simulink model "mcb_pmsm_foc_sensorless_f28379d"  (R2024b)
settings: Solver=FixedStepDiscrete  StartTime=0.0  StopTime=8  RelTol=1e-3  EnableMultiTasking=on
InitFcn:
  | mcb_pmsm_foc_sensorless_f28379d_datascript;
model workspace (MAT data in the model file):
  encoderResolution = 2000
  hallOffset = '0.5'
  indexOffset = 850
  polePairs = '4'
values from neighbouring files (symbols this model uses):
  acceleration = 10000/PU_System.N_base    [mcb_pmsm_foc_sensorless_f28069MLaunchPad_edit_datascript.m]    (also in mcb_pmsm_foc_sensorless_f28379d_datascript.m)
  dataType = 'single'    [mcb_pmsm_foc_sensorless_f28069MLaunchPad_edit_datascript.m]    (also in mcb_pmsm_foc_sensorless_f28379d_datascript.m)
  inverter = mcb_SetInverterParameters('BoostXL-DRV8305')    [mcb_pmsm_foc_sensorless_f28069MLaunchPad_edit_datascript.m]    (also in mcb_pmsm_foc_sensorless_f28379d_datascript.m = mcb_updateInverterParameters(pmsm,inverter,target))
  MAX_OL_NEG_SPD = -0.2    [mcb_pmsm_foc_sensorless_f28069MLaunchPad_edit_datascript.m]    (also in mcb_pmsm_foc_sensorless_f28379d_datascript.m)
  MAX_OL_POS_SPD = 0.2    [mcb_pmsm_foc_sensorless_f28069MLaunchPad_edit_datascript.m]    (also in mcb_pmsm_foc_sensorless_f28379d_datascript.m)
  MAX_OL_VD_LIMIT = 0.6    [mcb_pmsm_foc_sensorless_f28069MLaunchPad_edit_datascript.m]    (also in mcb_pmsm_foc_sensorless_f28379d_datascript.m)
  MIN_CL_NEG_SPD = -0.15    [mcb_pmsm_foc_sensorless_f28069MLaunchPad_edit_datascript.m]    (also in mcb_pmsm_foc_sensorless_f28379d_datascript.m)
  MIN_CL_POS_SPD = 0.15    [mcb_pmsm_foc_sensorless_f28069MLaunchPad_edit_datascript.m]    (also in mcb_pmsm_foc_sensorless_f28379d_datascript.m)
  MIN_OL_VD_LIMIT = 0.15    [mcb_pmsm_foc_sensorless_f28069MLaunchPad_edit_datascript.m]    (also in mcb_pmsm_foc_sensorless_f28379d_datascript.m)
  one_sec_tick = uint16(1/Ts_speed)    [mcb_pmsm_foc_sensorless_f28069MLaunchPad_edit_datascript.m]    (also in mcb_pmsm_foc_sensorless_f28379d_datascript.m)
  PI_params = mcb_SetControllerParameters(pmsm,inverter,PU_System,T_pwm,2*Ts,2*Ts_speed)    [mcb_pmsm_foc_sensorless_f28069MLaunchPad_edit_datascript.m]    (also in mcb_pmsm_foc_sensorless_f28379d_datascript.m)
  pmsm = mcb_SetPMSMMotorParameters('BLY172S')    [mcb_pmsm_foc_sensorless_f28069MLaunchPad_edit_datascript.m]    (also in mcb_pmsm_foc_sensorless_f28379d_datascript.m)
  PU_System = mcb_SetPUSystem(pmsm,inverter)    [mcb_pmsm_foc_sensorless_f28069MLaunchPad_edit_datascript.m]    (also in mcb_pmsm_foc_sensorless_f28379d_datascript.m)
  RAMP_STEP_SIZE = 0.001    [mcb_pmsm_foc_sensorless_f28069MLaunchPad_edit_datascript.m]    (also in mcb_pmsm_foc_sensorless_f28379d_datascript.m)
  Speed_openLoop_PU = 0.1    [mcb_pmsm_foc_sensorless_f28069MLaunchPad_edit_datascript.m]    (also in mcb_pmsm_foc_sensorless_f28379d_datascript.m)
  target = mcb_SetProcessorDetails('F28069M',PWM_frequency)    [mcb_pmsm_foc_sensorless_f28069MLaunchPad_edit_datascript.m]    (also in mcb_pmsm_foc_sensorless_f28379d_datascript.m = mcb_SetProcessorDetails('F28379D',PWM_frequency))
  Ts = T_pwm    (= 5e-05)    [mcb_pmsm_foc_sensorless_f28069MLaunchPad_edit_datascript.m]    (also in mcb_pmsm_foc_sensorless_f28379d_datascript.m)
  Ts_motor = T_pwm/2    (= 2.5e-05)    [mcb_pmsm_foc_sensorless_f28069MLaunchPad_edit_datascript.m]    (also in mcb_pmsm_foc_sensorless_f28379d_datascript.m)
  Ts_simulink = T_pwm/2    (= 2.5e-05)    [mcb_pmsm_foc_sensorless_f28069MLaunchPad_edit_datascript.m]    (also in mcb_pmsm_foc_sensorless_f28379d_datascript.m)
  Ts_speed = 10*Ts    (= 0.0005)    [mcb_pmsm_foc_sensorless_f28069MLaunchPad_edit_datascript.m]    (also in mcb_pmsm_foc_sensorless_f28379d_datascript.m)
  two_sec_tick = uint16(2/Ts_speed)    [mcb_pmsm_foc_sensorless_f28069MLaunchPad_edit_datascript.m]    (also in mcb_pmsm_foc_sensorless_f28379d_datascript.m)
undefined symbols (not defined in the file or in its folder): Down, GPTRIP1SEL, GPTRIP2SEL, TZ1, TZ2, Up
libraries: mcbcontrolslib x17, simulink x8, c2802xlib x7, c280xlib x5, c2837xDlib x4, slpidlib x3, mcbpositiondecoderlib x3, mcbsensorlessestimatorlib x2, svdschedulerlib x2, svdutilitieslib x1, mcbplantlib x1, autolibpmsmexterior x1
(part 3 of 3)

== system mcb_pmsm_foc_sensorless_f28379d/Hardware Init/Variant Subsystem/Code Generation/Calculate ADC Offset  ==
  Enable : EnablePort
  Constant : Constant  Value=8
  Constant1 : Constant  Value=inverter.CtSensOffsetMax  OutDataTypeStr=Inherit: Inherit via back propagation
  Constant2 : Constant  Value=inverter.CtSensOffsetMin  OutDataTypeStr=Inherit: Inherit via back propagation
  Divide : Product  Inputs=*/  OutDataTypeStr=uint16
  Divide1 : Product  Inputs=*/  OutDataTypeStr=uint16
  For Iterator Subsystem : Subsystem  TreatAsAtomicUnit=on
  If : If  NumInputs=3  IfExpression=u1 > u3 & u1 < u2
  If Action Subsystem : Subsystem  TreatAsAtomicUnit=on
  If Action Subsystem1 : Subsystem  TreatAsAtomicUnit=on
  If Action Subsystem2 : Subsystem  TreatAsAtomicUnit=on
  If Action Subsystem3 : Subsystem  TreatAsAtomicUnit=on
  If1 : If  NumInputs=3  IfExpression=u1 > u3 & u1 < u2
  wires:
  For Iterator Subsystem/2(Out2) -> Divide1/1
  Divide/1 -> If Action Subsystem/1(In1), If/1
  For Iterator Subsystem/1(Out1) -> Divide/1
  Constant/1 -> Divide1/2, Divide/2
  Divide1/1 -> If Action Subsystem2/1(In1), If1/1
  If/1 -> If Action Subsystem/Action
  If/2 -> If Action Subsystem1/Action
  If1/1 -> If Action Subsystem2/Action
  If1/2 -> If Action Subsystem3/Action
  Constant1/1 -> If1/2, If/2
  Constant2/1 -> If/3, If1/3

== system mcb_pmsm_foc_sensorless_f28379d/Hardware Init/Variant Subsystem/Code Generation/DRV Enable ==
  note: Enable inverter in CPU1
  In : Inport
  ADC Gain Setting : Subsystem
  Constant : Constant  Value=inverter.EnableLogic
  Digital Output : c2837xDlib/Digital Output  Priority=10  GPIO_Number=GPIO120~GPIO127  GPIO_Bit0=off  GPIO_BIT0_Toggle=off  GPIO_Bit1=off  GPIO_BIT1_Toggle=off  GPIO_Bit2=off  GPIO_BIT2_Toggle=off  GPIO_Bit3=off  GPIO_BIT3_Toggle=off  GPIO_Bit4=on  GPIO_BIT4_Toggle=off  GPIO_Bit5=off  GPIO_BIT5_Toggle=off  GPIO_Bit6=off  GPIO_BIT6_Toggle=off  GPIO_Bit7=off  GPIO_BIT7_Toggle=off
  Digital Output1 : c2837xDlib/Digital Output  Priority=10  GPIO_Number=GPIO16~GPIO23  GPIO_Bit0=off  GPIO_BIT0_Toggle=off  GPIO_Bit1=off  GPIO_BIT1_Toggle=off  GPIO_Bit2=off  GPIO_BIT2_Toggle=off  GPIO_Bit3=off  GPIO_BIT3_Toggle=off  GPIO_Bit4=off  GPIO_BIT4_Toggle=off  GPIO_Bit5=off  GPIO_BIT5_Toggle=off  GPIO_Bit6=on  GPIO_BIT6_Toggle=off  GPIO_Bit7=off  GPIO_BIT7_Toggle=off
  Inverter Enable : Constant  OutDataTypeStr=uint16  SampleTime=-1
  NOT : Logic  Operator=NOT  IconShape=distinctive  AllPortsSameDT=off  OutDataTypeStr=boolean
  RunTimeMeasurement : Constant  OutDataTypeStr=uint16  SampleTime=-1
  Switch : Switch  Criteria=u2 > Threshold  SaturateOnIntegerOverflow=off  InputSameDT=off
  wires:
  RunTimeMeasurement/1 -> Digital Output1/1
  NOT/1 -> Switch/3  "Active low logic for inverter enable"
  Inverter Enable/1 -> Switch/1, NOT/1  "Active high logic for inverter enable"
  Constant/1 -> ADC Gain Setting/Enable, Switch/2
  Switch/1 -> Digital Output/1
  In/1 -> ADC Gain Setting/1(In1)

== system mcb_pmsm_foc_sensorless_f28379d/Hardware Init/Variant Subsystem/Code Generation/Default ADC Offset ==
  Enable : EnablePort
  Constant : Constant  Value=inverter.CtSensAOffset  OutDataTypeStr=Inherit: Inherit via back propagation
  Constant1 : Constant  Value=inverter.CtSensBOffset  OutDataTypeStr=Inherit: Inherit via back propagation
  Data Store Write1 : DataStoreWrite  DataStoreName=IaOffset  IndexOptions=Index vector (dialog)  Indices=1  OutputSizes=1
  Data Store Write2 : DataStoreWrite  DataStoreName=IbOffset  IndexOptions=Index vector (dialog)  Indices=1  OutputSizes=1
  wires:
  Constant/1 -> Data Store Write1/1
  Constant1/1 -> Data Store Write2/1

== system mcb_pmsm_foc_sensorless_f28379d/Serial Receive/SCI_Rx/Code Generation/Data_Type_Fixed_Point ==
  SCI Receive : c280xlib/SCI Receive  sciModule=A  dataHead=''  headerCheckMaxCount=16  dataTail=''  dataType=uint32  dataLenOptions=Length via dialog  dataDim=2  maxDataLength=1  initValue=0  errOption=Output the last received value  errValue=0  sampleTime=-1  blockingMode=on  timeOut=0.00875  outputStatus=off
  Data : Outport
  wires:
  SCI Receive/1 -> Data/1

== system mcb_pmsm_foc_sensorless_f28379d/Serial Receive/SCI_Rx/Code Generation/Data_Type_Float ==
  SCI Receive : c280xlib/SCI Receive  sciModule=A  dataHead=''  headerCheckMaxCount=16  dataTail=''  dataType=single  dataLenOptions=Length via dialog  dataDim=2  maxDataLength=1  initValue=0  errOption=Output the last received value  errValue=0  sampleTime=-1  blockingMode=on  timeOut=0.00875  outputStatus=off
  Data : Outport
  wires:
  SCI Receive/1 -> Data/1

== system mcb_pmsm_foc_sensorless_f28379d/Serial Receive/SCI_Rx/Simulation/Data_Conditioning_Tx ==
  In1 : Inport
  In2 : Inport  Port=2
  Data_Type_Fixed_Point : Subsystem  VariantControl=~isequal(dataType, 'single')
  Data_Type_Float : Subsystem  VariantControl=isequal(dataType, 'single')
  Data : Outport

== system mcb_pmsm_foc_sensorless_f28379d/Serial Receive/SCI_Rx/Simulation/Parse ==
  Enable_PWM : Inport
  Debug_signals : Inport  Port=2
  Bitwise Operator : simulink/Logic and Bit Operations/Bitwise Operator  logicop=AND  UseBitMask=on  BitMask=hex2dec('0001')  BitMaskRealWorld=Stored Integer
  Bitwise Operator1 : simulink/Logic and Bit Operations/Bitwise Operator  logicop=AND  UseBitMask=on  BitMask=hex2dec('00F0')  BitMaskRealWorld=Stored Integer
  Shift Arithmetic1 : ArithShift  BitShiftNumber=-4
  Sum : Sum
  Data : Outport
  wires:
  Bitwise Operator/1 -> Sum/1
  Debug_signals/1 -> Shift Arithmetic1/1
  Sum/1 -> Data/1
  Shift Arithmetic1/1 -> Bitwise Operator1/1
  Enable_PWM/1 -> Bitwise Operator/1
  Bitwise Operator1/1 -> Sum/2

== system mcb_pmsm_foc_sensorless_f28379d/Current Control/Closed Loop/Open_Loop_Control/Accumulate1/Subsystem ==
  Input : Inport
  Enable : EnablePort
  Out1 : Outport  InitialOutput=0
  wires:
  Input/1 -> Out1/1

== system mcb_pmsm_foc_sensorless_f28379d/Current Control/Input Scaling/Calculate Phase Currents/Data_Type/Data_Type_Fixed_Point ==
  In1 : Inport
  Data Type Conversion : DataTypeConversion  OutDataTypeStr=fixdt(1,32,17)  ConvertRealWorld=Stored Integer (SI)  RndMeth=Simplest  SaturateOnIntegerOverflow=off
  Data Type Conversion1 : DataTypeConversion  OutDataTypeStr=dataType  RndMeth=Simplest  SaturateOnIntegerOverflow=off
  Q17 per unit conversion : ArithShift  BitShiftNumber=-6
  Iab_meas_PU : Outport
  wires:
  In1/1 -> Q17 per unit conversion/1
  Data Type Conversion1/1 -> Iab_meas_PU/1
  Data Type Conversion/1 -> Data Type Conversion1/1
  Q17 per unit conversion/1 -> Data Type Conversion/1

== system mcb_pmsm_foc_sensorless_f28379d/Current Control/Input Scaling/Calculate Phase Currents/Data_Type/Data_Type_Float ==
  In1 : Inport
  Get ADC Voltage : Gain  Gain=target.ADC_Vref /target.ADC_MaxCount  OutDataTypeStr=dataType  RndMeth=Simplest
  Get Currents : Gain  Gain=1/inverter.ISenseVoltPerAmp  RndMeth=Simplest  OutDataTypeStr=Inherit: Same as input
  PU_Conversion : Gain  Gain=1/PU_System.I_base  RndMeth=Simplest  OutDataTypeStr=Inherit: Same as input
  Iab_meas_PU : Outport
  wires:
  Get ADC Voltage/1 -> Get Currents/1
  Get Currents/1 -> PU_Conversion/1
  PU_Conversion/1 -> Iab_meas_PU/1
  In1/1 -> Get ADC Voltage/1

== system mcb_pmsm_foc_sensorless_f28379d/Current Control/Input Scaling/Calculate position and speed/Flux Observer/DC component removal ==
  SigIN : Inport
  IIR Filter : mcbcontrolslib/IIR Filter  VariantControl=Low Pass Filter  VariantSelect=High-pass  FilterConstantInputType=Specify via dialog  Filter_constant=0.0005*(Ts/50e-6)  advancedSettings=on  Ts=50e-6  cutOff_freq=1
  SigOUT : Outport
  wires:
  SigIN/1 -> IIR Filter/1
  IIR Filter/1 -> SigOUT/1

== system mcb_pmsm_foc_sensorless_f28379d/Current Control/Input Scaling/Calculate position and speed/Flux Observer/DC component removal1 ==
  SigIN : Inport
  IIR Filter : mcbcontrolslib/IIR Filter  VariantControl=Low Pass Filter  VariantSelect=Low-pass  FilterConstantInputType=Specify via dialog  Filter_constant=0.005*(Ts/50e-6)  advancedSettings=on  Ts=50e-6  cutOff_freq=1
  Sum6 : Sum  Inputs=|+-  RndMeth=Simplest  OutDataTypeStr=Inherit: Same as first input
  SigOUT : Outport
  wires:
  Sum6/1 -> SigOUT/1
  SigIN/1 -> Sum6/1, IIR Filter/1
  IIR Filter/1 -> Sum6/2

== system mcb_pmsm_foc_sensorless_f28379d/Current Control/SCI_Tx/Code Generation/Data_Conditioning_Tx/Data_Type_Fixed_Point ==
  In1 : Inport
  Data Type Conversion : DataTypeConversion  OutDataTypeStr=fixdt(1,32,28)  RndMeth=Simplest  SaturateOnIntegerOverflow=off
  Data Type Conversion3 : DataTypeConversion  OutDataTypeStr=uint32  ConvertRealWorld=Stored Integer (SI)  RndMeth=Simplest  SaturateOnIntegerOverflow=off
  Data_Log : Outport
  wires:
  In1/1 -> Data Type Conversion/1
  Data Type Conversion3/1 -> Data_Log/1
  Data Type Conversion/1 -> Data Type Conversion3/1

== system mcb_pmsm_foc_sensorless_f28379d/Current Control/SCI_Tx/Code Generation/Data_Conditioning_Tx/Data_Type_Float ==
  In1 : Inport
  Byte Pack : svdutilitieslib/Byte Pack  maskPackedDataType=uint32  datatypes={'single'}  byteAlign=4  blockPlatform=tic2000
  Data_Log : Outport
  wires:
  Byte Pack/1 -> Data_Log/1
  In1/1 -> Byte Pack/1

== system mcb_pmsm_foc_sensorless_f28379d/Current Control/SCI_Tx/Code Generation/Data_Logging/Data ==
  Data : Inport
  Data_width : Inport  Port=2
  Action Port : ActionPort  ActionPortLabel=else
  Dummy : Constant  Value=hex2dec('0000')  OutDataTypeStr=uint32
  Mux : Mux  Inputs=2
  Data_out : Outport  VectorParamsAs1DForOutWhenUnconnected=off
  Iteration : Outport  Port=2  VectorParamsAs1DForOutWhenUnconnected=off
  wires:
  Data_width/1 -> Iteration/1
  Data/1 -> Mux/1
  Dummy/1 -> Mux/2
  Mux/1 -> Data_out/1

== system mcb_pmsm_foc_sensorless_f28379d/Current Control/SCI_Tx/Code Generation/Data_Logging/End ==
  Data : Inport
  Data_width : Inport  Port=2
  Action Port : ActionPort  ActionPortLabel=elseif(u1 == 599)
  Bias : Bias  Bias=1  SaturateOnIntegerOverflow=off
  End : Constant  Value=hex2dec('45454545')  OutDataTypeStr=uint32
  Mux : Mux  Inputs=2
  Data_out : Outport  VectorParamsAs1DForOutWhenUnconnected=off
  Iteration : Outport  Port=2  VectorParamsAs1DForOutWhenUnconnected=off
  wires:
  Data/1 -> Mux/1
  Data_width/1 -> Bias/1
  Bias/1 -> Iteration/1
  End/1 -> Mux/2
  Mux/1 -> Data_out/1

== system mcb_pmsm_foc_sensorless_f28379d/Current Control/SCI_Tx/Code Generation/Data_Logging/Start ==
  Data : Inport
  Data_width : Inport  Port=2
  Action Port : ActionPort  ActionPortLabel=if(u1 == 0)
  Bias : Bias  Bias=1  SaturateOnIntegerOverflow=off
  Mux : Mux  Inputs=2
  Start : Constant  Value=hex2dec('53535353')  OutDataTypeStr=uint32
  Data_out : Outport  VectorParamsAs1DForOutWhenUnconnected=off
  Iteration : Outport  Port=2  VectorParamsAs1DForOutWhenUnconnected=off
  wires:
  Data/1 -> Mux/2
  Data_width/1 -> Bias/1
  Bias/1 -> Iteration/1
  Start/1 -> Mux/1
  Mux/1 -> Data_out/1

== system mcb_pmsm_foc_sensorless_f28379d/Hardware Init/Variant Subsystem/Code Generation/Calculate ADC Offset /For Iterator Subsystem ==
  ADC_B2 : c2802xlib/ADC  Priority=20  blkParamProc=C2000_Type4  ADCModule=B  samplingMode=Single sample mode  ADCResolution=12-bit (Single-ended input)  useSOC1=SOC2  useSOC2=SOC0_SOC1  SOCAcquisitionWindow=15  SOCTriggerSource=Software  SOCInterruptTrigger=No ADCINT  Ts=-1  dType=uint16  postInterrupt=off  interruptSel=ADCINT1  ADCINTContinuous=on  endma=off  chdma=1  conv1=ADCINA0  conv2=ADCINA0 and ADCINB0  conv1_Type4=ADCIN2  conv2_Type4=ADCIN0 and ADCIN1
  ADC_C2 : c2802xlib/ADC  Priority=20  blkParamProc=C2000_Type4  ADCModule=C  samplingMode=Single sample mode  ADCResolution=12-bit (Single-ended input)  useSOC1=SOC2  useSOC2=SOC0_SOC1  SOCAcquisitionWindow=15  SOCTriggerSource=Software  SOCInterruptTrigger=No ADCINT  Ts=-1  dType=uint16  postInterrupt=off  interruptSel=ADCINT1  ADCINTContinuous=on  endma=off  chdma=1  conv1=ADCINA0  conv2=ADCINA0 and ADCINB0  conv1_Type4=ADCIN2  conv2_Type4=ADCIN0 and ADCIN1
  For Iterator : ForIterator  IterationLimit=16  IterationVariableDataType=uint16
  If : If  IfExpression=u1 > 8  ShowElse=off
  If Action Subsystem : Subsystem  TreatAsAtomicUnit=on
  Out1 : Outport
  Out2 : Outport  Port=2
  wires:
  For Iterator/1 -> If/1
  ADC_C2/1 -> If Action Subsystem/1(In1)
  ADC_B2/1 -> If Action Subsystem/2(In2)
  If Action Subsystem/1(Out1) -> Out1/1
  If Action Subsystem/2(Out2) -> Out2/1
  If/1 -> If Action Subsystem/Action

== system mcb_pmsm_foc_sensorless_f28379d/Hardware Init/Variant Subsystem/Code Generation/Calculate ADC Offset /If Action Subsystem ==
  In1 : Inport
  Action Port : ActionPort  ActionPortLabel=if(u1 > u3 & u1 < u2)
  Data Store Write1 : DataStoreWrite  DataStoreName=IaOffset  IndexOptions=Index vector (dialog)  Indices=1  OutputSizes=1
  wires:
  In1/1 -> Data Store Write1/1

== system mcb_pmsm_foc_sensorless_f28379d/Hardware Init/Variant Subsystem/Code Generation/Calculate ADC Offset /If Action Subsystem1 ==
  Action Port : ActionPort  ActionPortLabel=else
  Constant : Constant  Value=inverter.CtSensAOffset  OutDataTypeStr=Inherit: Inherit via back propagation
  Data Store Write1 : DataStoreWrite  DataStoreName=IaOffset  IndexOptions=Index vector (dialog)  Indices=1  OutputSizes=1
  wires:
  Constant/1 -> Data Store Write1/1

== system mcb_pmsm_foc_sensorless_f28379d/Hardware Init/Variant Subsystem/Code Generation/Calculate ADC Offset /If Action Subsystem2 ==
  In1 : Inport
  Action Port : ActionPort  ActionPortLabel=if(u1 > u3 & u1 < u2)
  Data Store Write2 : DataStoreWrite  DataStoreName=IbOffset  IndexOptions=Index vector (dialog)  Indices=1  OutputSizes=1
  wires:
  In1/1 -> Data Store Write2/1

== system mcb_pmsm_foc_sensorless_f28379d/Hardware Init/Variant Subsystem/Code Generation/Calculate ADC Offset /If Action Subsystem3 ==
  Action Port : ActionPort  ActionPortLabel=else
  Constant1 : Constant  Value=inverter.CtSensBOffset  OutDataTypeStr=Inherit: Inherit via back propagation
  Data Store Write2 : DataStoreWrite  DataStoreName=IbOffset  IndexOptions=Index vector (dialog)  Indices=1  OutputSizes=1
  wires:
  Constant1/1 -> Data Store Write2/1

== system mcb_pmsm_foc_sensorless_f28379d/Hardware Init/Variant Subsystem/Code Generation/DRV Enable/ADC Gain Setting ==
  In1 : Inport
  Enable : EnablePort
  Demux : Demux  Outputs=2
  Display : Display
      settings: Format=hex (Stored Integer)
  Display1 : Display
      settings: Format=hex (Stored Integer)
  SPI Master Transfer : c280xlib/SPI Controller Transfer  SPISelect=SPI_A  ClockPolarity=Rising_edge  ClockPhase=No_delay  SPIModule=uint32(0)  Mode=Master  BusSpeed=uint32(1000000)  FirstBitToTransfer=Most significant bit (MSB)  ClockMode=0  BlockFunction=Transfer  EnableRegisterAddress=off  RegisterAddress=0  OutputDataType=int8  OutputDataLength=1  DataBits=16  UseCustomSSPin=Provided by the SPI peripheral  ActiveLowSSPin=Active low  Pin=61
  SPI Master Transfer1 : c280xlib/SPI Controller Transfer  SPISelect=SPI_A  ClockPolarity=Rising_edge  ClockPhase=No_delay  SPIModule=uint32(0)  Mode=Master  BusSpeed=uint32(1000000)  FirstBitToTransfer=Most significant bit (MSB)  ClockMode=0  BlockFunction=Transfer  EnableRegisterAddress=off  RegisterAddress=0  OutputDataType=int8  OutputDataLength=1  DataBits=16  UseCustomSSPin=Provided by the SPI peripheral  ActiveLowSSPin=Active low  Pin=61
  wires:
  Demux/2 -> SPI Master Transfer1/1
  SPI Master Transfer/1 -> Display/1
  SPI Master Transfer1/1 -> Display1/1
  Demux/1 -> SPI Master Transfer/1
  In1/1 -> Demux/1

== system mcb_pmsm_foc_sensorless_f28379d/Serial Receive/SCI_Rx/Simulation/Data_Conditioning_Tx/Data_Type_Fixed_Point ==
  In1 : Inport
  In2 : Inport  Port=2
  Data Type Conversion : DataTypeConversion  OutDataTypeStr=fixdt(1,32,28)  RndMeth=Simplest  SaturateOnIntegerOverflow=off
  Data Type Conversion1 : DataTypeConversion  OutDataTypeStr=uint32  RndMeth=Simplest  SaturateOnIntegerOverflow=off
  Data Type Conversion3 : DataTypeConversion  OutDataTypeStr=uint32  ConvertRealWorld=Stored Integer (SI)  RndMeth=Simplest  SaturateOnIntegerOverflow=off
  Mux : Mux  Inputs=2
  Data : Outport
  wires:
  In1/1 -> Data Type Conversion/1
  Data Type Conversion3/1 -> Mux/1
  Data Type Conversion/1 -> Data Type Conversion3/1
  In2/1 -> Data Type Conversion1/1
  Data Type Conversion1/1 -> Mux/2
  Mux/1 -> Data/1

== system mcb_pmsm_foc_sensorless_f28379d/Serial Receive/SCI_Rx/Simulation/Data_Conditioning_Tx/Data_Type_Float ==
  In1 : Inport
  In2 : Inport  Port=2
  Data Type Conversion2 : DataTypeConversion  OutDataTypeStr=single  RndMeth=Simplest  SaturateOnIntegerOverflow=off
  Mux : Mux  Inputs=2
  Data : Outport
  wires:
  In1/1 -> Mux/1
  Mux/1 -> Data/1
  In2/1 -> Data Type Conversion2/1
  Data Type Conversion2/1 -> Mux/2

== system mcb_pmsm_foc_sensorless_f28379d/Hardware Init/Variant Subsystem/Code Generation/Calculate ADC Offset /For Iterator Subsystem/If Action Subsystem ==
  In1 : Inport
  In2 : Inport  Port=2
  Action Port : ActionPort  ActionPortLabel=if(u1 > 8)
  Memory : Memory  InheritSampleTime=on
  Memory1 : Memory  InheritSampleTime=on
  Sum : Sum
  Sum1 : Sum
  Out1 : Outport
  Out2 : Outport  Port=2
  wires:
  In1/1 -> Sum/1
  Sum/1 -> Out1/1, Memory/1
  In2/1 -> Sum1/1
  Memory/1 -> Sum/2
  Sum1/1 -> Out2/1, Memory1/1
  Memory1/1 -> Sum1/2

== stateflow chart mcb_pmsm_foc_sensorless_f28379d/State Machine Handler/State Machine OL - CL ==
  state RunMode
    state PositiveSpeedRun
      state OpenLoopPosRun
        during:
        if(SpdCmd>MAX_OL_POS_SPD)
        SpdRef=MAX_OL_POS_SPD;
        else
        SpdRef=SpdCmd;
        end
      state PreparePosCLSwitch
        entry:
        Id0_out=Id0_in;
        SpdRef=MAX_OL_POS_SPD;
      state TransferToPosClosedLoop
        entry:
        EnClosedLoop=true;
        Id0_out=Id0_in;
        during:
        Id0_out = ComputeId0(Id0_out,RAMP_STEP_SIZE);
      state TransferToOpenLoop
        entry:
        SpdRef=MAX_OL_POS_SPD*1.03;
      state ClosedLoopPosRun
        entry:
        SpdRef=SpdCmd;
        Id0_out=0;
        during:
        SpdRef=SpdCmd;
      (junction 118) -> (junction 94) [order 1] : [SpdCmd>MAX_OL_POS_SPD]
      (junction 94) -> PreparePosCLSwitch [order 2] : [SpdRef<MAX_OL_POS_SPD]
      (junction 94) -> TransferToPosClosedLoop [order 1] : [SpdRef>=MAX_OL_POS_SPD]
      OpenLoopPosRun -> (junction 118)
      PreparePosCLSwitch -> TransferToPosClosedLoop : after(one_sec_tick,tick)
      TransferToPosClosedLoop -> ClosedLoopPosRun : after(two_sec_tick,tick)[Id0_out<=RAMP_STEP_SIZE]
      ClosedLoopPosRun -> TransferToOpenLoop : [SpdCmd<MIN_CL_POS_SPD]
    state InitOpenLoopRun
      entry:
      Enable=true;
      EnClosedLoop=false;
      during:
      if(SpdCmd>MAX_OL_POS_SPD)
      SpdRef=MAX_OL_POS_SPD;
      elseif (SpdCmd<MAX_OL_NEG_SPD)
      SpdRef=MAX_OL_NEG_SPD;
      else
      SpdRef=SpdCmd;
      end
      Id0_out=Id0_in;
    state Id0_out = ComputeId0(Id0_in,RAMP_STEP_SIZE) [function]
    state NegativeSpeedRun
      state OpenLoopNegRun
        during:
        if(SpdCmd<MAX_OL_NEG_SPD)
        SpdRef=MAX_OL_NEG_SPD;
        else
        SpdRef=SpdCmd;
        end
      state TransferToNegClosedLoop
        entry:
        EnClosedLoop=true;
        Id0_out=Id0_in;
        during:
        Id0_out = ComputeId0(Id0_out,RAMP_STEP_SIZE);
      state PrepareNegCLSwitch
        entry:
        Id0_out=Id0_in;
        SpdRef=MAX_OL_NEG_SPD;
      state TransferToOpenLoop_NEG
        entry:
        SpdRef=MAX_OL_NEG_SPD*1.03;
      state ClosedLoopRun_NEG
        entry:
        SpdRef=SpdCmd;
        Id0_out=0;
        during:
        SpdRef=SpdCmd;
      OpenLoopNegRun -> (junction 121)
      (junction 121) -> (junction 124) [order 2] : [SpdCmd<MAX_OL_NEG_SPD]
      (junction 124) -> TransferToNegClosedLoop [order 2] : [SpdRef<=MAX_OL_NEG_SPD]
      (junction 124) -> PrepareNegCLSwitch [order 1] : [SpdRef>MAX_OL_NEG_SPD]
      PrepareNegCLSwitch -> TransferToNegClosedLoop : after(one_sec_tick,tick)
      TransferToNegClosedLoop -> ClosedLoopRun_NEG : after(two_sec_tick,tick)[Id0_out<=RAMP_STEP_SIZE]
      ClosedLoopRun_NEG -> TransferToOpenLoop_NEG : [SpdCmd>MIN_CL_NEG_SPD]
    InitOpenLoopRun -> OpenLoopPosRun [order 1] : [SpdCmd > 0]
    (junction 118) -> OpenLoopNegRun [order 2] : [SpdCmd<0]
    (junction 121) -> OpenLoopPosRun [order 1] : [SpdCmd>0]
    (default) -> InitOpenLoopRun
    TransferToOpenLoop_NEG -> InitOpenLoopRun : after(one_sec_tick,tick)
    InitOpenLoopRun -> OpenLoopNegRun [order 2] : [SpdCmd<0]
    TransferToOpenLoop -> InitOpenLoopRun : after(one_sec_tick,tick)
  state Halt
    entry:
    Enable=false;
    SpdRef=0;
    EnClosedLoop=false;
  Halt -> RunMode : [Start==true && SpdCmd~=0]
  (default) -> Halt
  RunMode -> Halt : [Start==false || SpdCmd==0]
  data: Id0_in function_input dataType size=1; RAMP_STEP_SIZE function_input dataType size=1; Id0_out function_output; Enable output; EnClosedLoop output; SpdRef output; Start input; SpdCmd input; Id0_out output dataType; Id0_in input; one_sec_tick parameter; two_sec_tick parameter; RAMP_STEP_SIZE parameter dataType; MAX_OL_NEG_SPD parameter dataType; MIN_CL_NEG_SPD parameter dataType; MIN_CL_POS_SPD parameter dataType; MAX_OL_POS_SPD parameter dataType
